simulink model "testTurtleBotModel"  (R2019b)
settings: Solver=FixedStepAuto  StartTime=0.0  StopTime=inf  FixedStep=sampleTime  RelTol=1e-3
PreLoadFcn:
  | linVel = 0;
  | angVel = 0;
  | sampleTime = 0.25;
  | connectToRobot;
InitFcn:
  | close all;
model workspace (MAT data in the model file):
  SL_ROS_VariableLengthArrays_MaxSizes.CommonInfo.ArrayTruncateAction = 'EmitWarning'
  SL_ROS_VariableLengthArrays_MaxSizes.MsgTypeMap = containers.Map
  SL_ROS_VariableLengthArrays_MaxSizes.MsgTypeMap.serialization.keys = {'sensor_msgs/CompressedImage', 'sensor_msgs/Image', 'sensor_msgs/LaserScan', 'sensor_msgs/PointCloud2'}
  SL_ROS_VariableLengthArrays_MaxSizes.MsgTypeMap.serialization.values{1}(1).PropertyName = 'Data'
  SL_ROS_VariableLengthArrays_MaxSizes.MsgTypeMap.serialization.values{1}(1).DataType = 'uint8'
  SL_ROS_VariableLengthArrays_MaxSizes.MsgTypeMap.serialization.values{1}(1).MaxLength = 6220800
  SL_ROS_VariableLengthArrays_MaxSizes.MsgTypeMap.serialization.values{1}(2).PropertyName = 'Format'
  SL_ROS_VariableLengthArrays_MaxSizes.MsgTypeMap.serialization.values{1}(2).DataType = 'uint8'
  SL_ROS_VariableLengthArrays_MaxSizes.MsgTypeMap.serialization.values{1}(2).MaxLength = 128
  SL_ROS_VariableLengthArrays_MaxSizes.MsgTypeMap.serialization.values{2}(1).PropertyName = 'Data'
  SL_ROS_VariableLengthArrays_MaxSizes.MsgTypeMap.serialization.values{2}(1).DataType = 'uint8'
  SL_ROS_VariableLengthArrays_MaxSizes.MsgTypeMap.serialization.values{2}(1).MaxLength = 921600
  SL_ROS_VariableLengthArrays_MaxSizes.MsgTypeMap.serialization.values{2}(2).PropertyName = 'Encoding'
  SL_ROS_VariableLengthArrays_MaxSizes.MsgTypeMap.serialization.values{2}(2).DataType = 'uint8'
  SL_ROS_VariableLengthArrays_MaxSizes.MsgTypeMap.serialization.values{2}(2).MaxLength = 128
  SL_ROS_VariableLengthArrays_MaxSizes.MsgTypeMap.serialization.values{3}(1).PropertyName = 'Intensities'
  SL_ROS_VariableLengthArrays_MaxSizes.MsgTypeMap.serialization.values{3}(1).DataType = 'single'
  SL_ROS_VariableLengthArrays_MaxSizes.MsgTypeMap.serialization.values{3}(1).MaxLength = 640
  SL_ROS_VariableLengthArrays_MaxSizes.MsgTypeMap.serialization.values{3}(2).PropertyName = 'Ranges'
  SL_ROS_VariableLengthArrays_MaxSizes.MsgTypeMap.serialization.values{3}(2).DataType = 'single'
  SL_ROS_VariableLengthArrays_MaxSizes.MsgTypeMap.serialization.values{3}(2).MaxLength = 640
  SL_ROS_VariableLengthArrays_MaxSizes.MsgTypeMap.serialization.values{4}(1).PropertyName = 'Data'
  SL_ROS_VariableLengthArrays_MaxSizes.MsgTypeMap.serialization.values{4}(1).DataType = 'uint8'
  SL_ROS_VariableLengthArrays_MaxSizes.MsgTypeMap.serialization.values{4}(1).MaxLength = 66355200
  SL_ROS_VariableLengthArrays_MaxSizes.MsgTypeMap.serialization.values{4}(2).PropertyName = 'Fields'
  SL_ROS_VariableLengthArrays_MaxSizes.MsgTypeMap.serialization.values{4}(2).DataType = 'sensor_msgs/PointField'
  SL_ROS_VariableLengthArrays_MaxSizes.MsgTypeMap.serialization.values{4}(2).MaxLength = 16
  SL_ROS_VariableLengthArrays_MaxSizes.MsgTypeMap.serialization.uniformity = 0
  SL_ROS_VariableLengthArrays_MaxSizes.MsgTypeMap.serialization.keyType = 'char'
  SL_ROS_VariableLengthArrays_MaxSizes.MsgTypeMap.serialization.valueType = 'any'
undefined symbols (not defined in the file or in its folder): Angular, Linear
libraries: robotlib x8, robotcorelib x1, visionsinks x1
settings Model: EnablePacing=on  Creator=scastro  LastModifiedBy=scastro
settings SolverCC: AutoInsertRateTranBlk=on
settings DataIOCC: ReturnWorkspaceOutputs=off
settings OptimizationCC: EnhancedBackFolding=on  PassReuseOutputArgsAs=Individual arguments  ZeroExternalMemoryAtStartup=off  ZeroInternalMemoryAtStartup=off  MaxStackSize=64  OptimizeBlockOrder=speed  DifferentSizesBufferReuse=on  OptimizationCustomize=off  EfficientTunableParamExpr=on
settings DebuggingCC: ParameterTunabilityLossMsg=error  ArithmeticOperatorsInVariantConditions=warning
settings HardwareCC: ProdBitPerPointer=32  ProdBitPerSizeT=32  ProdBitPerPtrDiffT=32  ProdLargestAtomicFloat=None  ProdIntDivRoundTo=Undefined  ProdEndianess=Unspecified  ProdWordSize=32  ProdHWDeviceType=Generic->Unspecified (assume 32-bit Generic)
settings SFSimCC: SimUseLocalCustomCode=off  MATLABDynamicMemAlloc=off  CustomCodeUndefinedFunction=UseInterfaceOnly
settings RTWCC: SystemTargetFile=ert.tlc  HardwareBoard=Robot Operating System (ROS)  TLCOptions="-aInlineSetEventsForThisBaseRateFcn=TLC_FALSE -aSuppressMultiTaskScheduler=TLC_FALSE  -aRateBasedStepFcn=0"  TemplateMakefile=ert_default_tmf  GenerateReport=on  RTWUseLocalCustomCode=off  Toolchain=Catkin  IncludeHyperlinkInReport=on  LaunchReport=on  TargetLang=C++  GenerateTraceInfo=on  GenerateTraceReport=on  GenerateTraceReportSl=on  GenerateTraceReportSf=on  GenerateTraceReportEml=on
settings CodeAppCC: ForceParamTrailComments=on  IgnoreCustomStorageClasses=off  OperatorAnnotations=on  SimulinkDataObjDesc=on  SFDataObjDesc=on  InsertBlockDesc=on

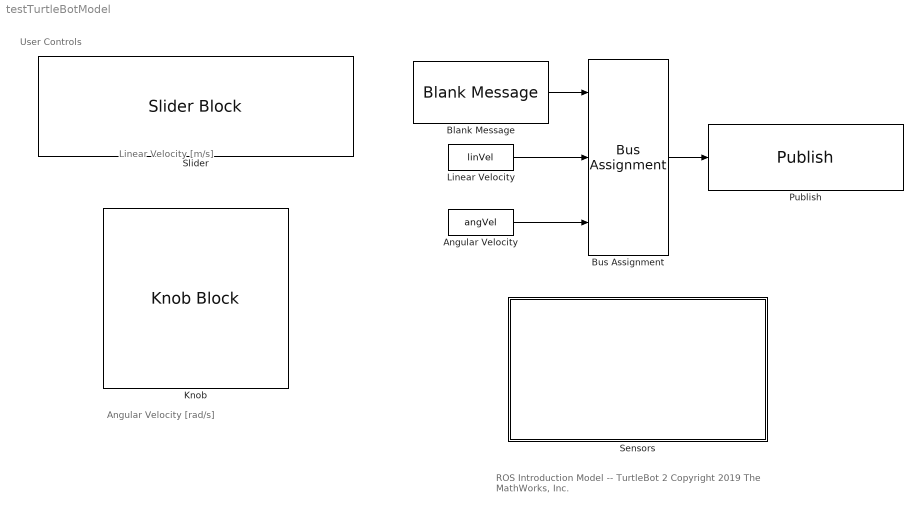
== system testTurtleBotModel ==
  note: User Controls
  note: Linear Velocity [m/s]
  note: Angular Velocity [rad/s]
  note: ROS Introduction Model -- TurtleBot 2
      |
      | Copyright 2019 The MathWorks, Inc.
  Angular Velocity : Constant  Value=angVel
  Blank Message : robotlib/Blank Message  messageClass=Message  entityType=geometry_msgs/Twist  messageType=geometry_msgs/Twist  SampleTime=-1
      settings: SourceProductBaseCode=RO
  Bus Assignment : BusAssignment  AssignedSignals=Linear.X,Angular.Z
  Knob : KnobBlock  ScaleMin=-1  ScaleMax=1  TickInterval=0.25
  Linear Velocity : Constant  Value=linVel
  Publish : robotlib/Publish  topicSource=Select from ROS network  topic=/mobile_base/commands/velocity  messageType=geometry_msgs/Twist  messageQueueLength=1
      settings: SourceProductBaseCode=RO
  Sensors : Subsystem
  Slider : SliderBlock  ScaleMin=-1  ScaleMax=1  TickInterval=0.25
  wires:
  Blank Message/1 -> Bus Assignment/1
  Bus Assignment/1 -> Publish/1
  Linear Velocity/1 -> Bus Assignment/2
  Angular Velocity/1 -> Bus Assignment/3

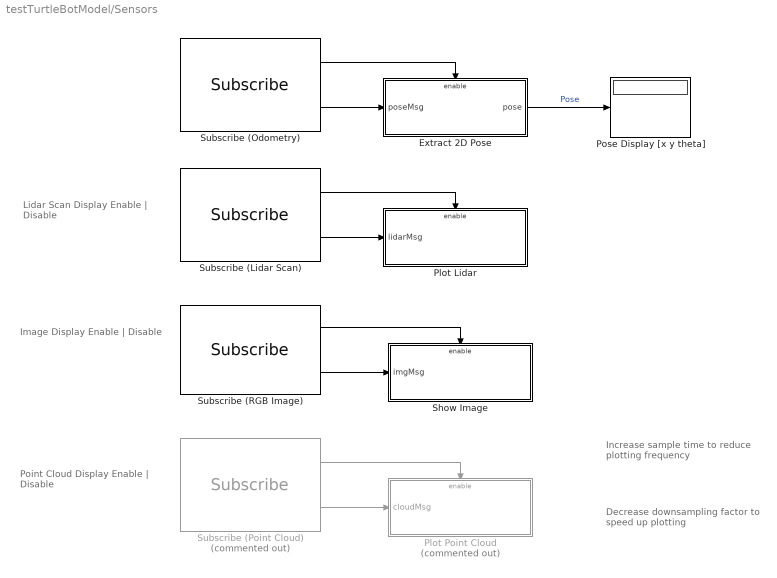
== system testTurtleBotModel/Sensors ==
  note: Increase sample time to reduce plotting frequency
  note: Lidar Scan Display
      | Enable | Disable
  note: Image Display
      | Enable | Disable
  note: Point Cloud Display
      | Enable | Disable
  note: Decrease downsampling factor to speed up plotting
  Extract 2D Pose : Subsystem  TreatAsAtomicUnit=on
  Plot Lidar : Subsystem  TreatAsAtomicUnit=on
  Plot Point Cloud : Subsystem  Commented=on  TreatAsAtomicUnit=on
  Pose Display [x y theta] : Display
  Show Image : Subsystem  TreatAsAtomicUnit=on
  Subscribe (Lidar Scan) : robotlib/Subscribe  topicSource=Select from ROS network  topic=/scan  messageType=sensor_msgs/LaserScan  sampleTime=-1  messageQueueLength=1
      settings: SourceProductBaseCode=RO
  Subscribe (Odometry) : robotlib/Subscribe  topicSource=Select from ROS network  topic=/odom  messageType=nav_msgs/Odometry  sampleTime=-1  messageQueueLength=1
      settings: SourceProductBaseCode=RO
  Subscribe (Point Cloud) : robotlib/Subscribe  Commented=on  topicSource=Select from ROS network  topic=/camera/depth/points  messageType=sensor_msgs/PointCloud2  sampleTime=5  messageQueueLength=1
      settings: SourceProductBaseCode=RO
  Subscribe (RGB Image) : robotlib/Subscribe  topicSource=Select from ROS network  topic=/camera/rgb/image_color  messageType=sensor_msgs/Image  sampleTime=-1  messageQueueLength=1
      settings: SourceProductBaseCode=RO
  wires:
  Extract 2D Pose/1(pose) -> Pose Display [x y theta]/1  "Pose"
  Subscribe (Odometry)/1 -> Extract 2D Pose/Enable
  Subscribe (Odometry)/2 -> Extract 2D Pose/1(poseMsg)
  Subscribe (RGB Image)/2 -> Show Image/1(imgMsg)
  Subscribe (RGB Image)/1 -> Show Image/Enable
  Subscribe (Point Cloud)/2 -> Plot Point Cloud/1(cloudMsg)
  Subscribe (Point Cloud)/1 -> Plot Point Cloud/Enable
  Subscribe (Lidar Scan)/2 -> Plot Lidar/1(lidarMsg)
  Subscribe (Lidar Scan)/1 -> Plot Lidar/Enable

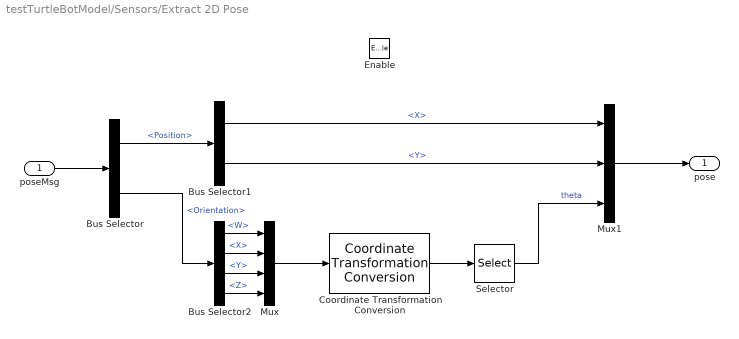
== system testTurtleBotModel/Sensors/Extract 2D Pose ==
  poseMsg : Inport
  Enable : EnablePort
  Bus Selector : BusSelector  OutputSignals=Pose.Pose.Position,Pose.Pose.Orientation
  Bus Selector1 : BusSelector  OutputSignals=X,Y
  Bus Selector2 : BusSelector  OutputSignals=W,X,Y,Z
  Coordinate Transformation Conversion : robotcorelib/Coordinate Transformation Conversion  InputRepresentation=Quaternion  InputEulerSequence=ZYX  ShowTrVecInputPort=on  OutputRepresentation=Euler Angles  OutputEulerSequence=ZYX  ShowTrVecOutputPort=on  SimulateUsing=Interpreted execution
      settings: SourceProductBaseCode=RO
  Mux : Mux
  Mux1 : Mux  Inputs=3
  Selector : Selector  InputPortWidth=3  IndexOptions=Index vector (dialog)  Indices=1  OutputSizes=1
  pose : Outport  VectorParamsAs1DForOutWhenUnconnected=off
  wires:
  poseMsg/1 -> Bus Selector/1
  Bus Selector/1 -> Bus Selector1/1  "<Position>"
  Bus Selector/2 -> Bus Selector2/1  "<Orientation>"
  Bus Selector2/1 -> Mux/1  "<W>"
  Bus Selector2/2 -> Mux/2  "<X>"
  Bus Selector2/3 -> Mux/3  "<Y>"
  Bus Selector2/4 -> Mux/4  "<Z>"
  Coordinate Transformation Conversion/1 -> Selector/1
  Mux/1 -> Coordinate Transformation Conversion/1
  Mux1/1 -> pose/1
  Selector/1 -> Mux1/3  "theta"
  Bus Selector1/2 -> Mux1/2  "<Y>"
  Bus Selector1/1 -> Mux1/1  "<X>"

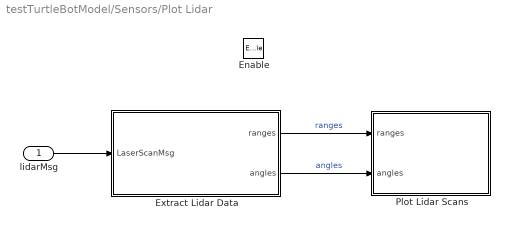
== system testTurtleBotModel/Sensors/Plot Lidar ==
  lidarMsg : Inport
  Enable : EnablePort  PropagateVarSize=During execution
  Extract Lidar Data : MATLAB Function  TreatAsAtomicUnit=on  mask(Extract Range Data){angLimits=[-pi/2 pi/2], rangeLimits=[0 5], numScans=640}
      mask prompts: angLimits "Min and Max Angles [rad]"; rangeLimits "Min and Max Ranges [m]"; numScans "Maximum Number of Scans"
  Plot Lidar Scans : MATLAB Function  InitFcn=clear lidarPlotHelper  TreatAsAtomicUnit=on
  wires:
  lidarMsg/1 -> Extract Lidar Data/1(LaserScanMsg)
  Extract Lidar Data/2(angles) -> Plot Lidar Scans/2(angles)  "angles"
  Extract Lidar Data/1(ranges) -> Plot Lidar Scans/1(ranges)  "ranges"

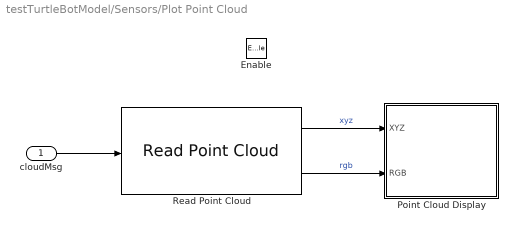
== system testTurtleBotModel/Sensors/Plot Point Cloud ==
  cloudMsg : Inport
  Enable : EnablePort
  Point Cloud Display : MATLAB Function  TreatAsAtomicUnit=on  mask(Point Cloud Display){xLim=[-2 2], yLim=[-0.5 2], zLim=[-0.5 5], sampleFactor=0.02}
      mask prompts: xLim "X Limits [m]"; yLim "Y Limits [m]"; zLim "Z Limits [m]"; sampleFactor "Downsample Factor"
      mask help: Displays a point cloud using the Computer Vision System Toolbox "pcplayer"
  Read Point Cloud : robotlib/Read Point Cloud  MaximumPointCloudSize=[1080, 1920]  PreserveStructure=off  ShowRGBOutput=on  ShowIntensityOutput=off  ShowErrorCodeOutput=off  VariableSizeOutputs=off
      settings: SourceProductName=Robotics System Toolbox  SourceProductBaseCode=RO
  wires:
  cloudMsg/1 -> Read Point Cloud/1
  Read Point Cloud/1 -> Point Cloud Display/1(XYZ)  "xyz"
  Read Point Cloud/2 -> Point Cloud Display/2(RGB)  "rgb"

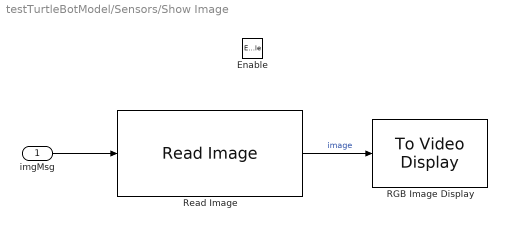
== system testTurtleBotModel/Sensors/Show Image ==
  imgMsg : Inport
  Enable : EnablePort
  RGB Image Display : visionsinks/To Video Display  windowSizeMode=Normal  openAtMdlStart=on  fullScreen=off  videoWindowX=1036  videoWindowY=102  saveWindowSize=off  videoWindowWidth=689  videoWindowHeight=510  inputColorFormat=RGB  inputType=Obsolete  imagePorts=One multidimensional signal  OutputDevice=On-screen video monitor  dataOrg=Column-major  isWindowOpen=off
      settings: SourceProductName=Computer Vision Toolbox
  Read Image : robotlib/Read Image  MaximumImageSize=[480, 640]  ImageEncoding=bgr8  ShowAlphaOutput=off  ShowErrorCodeOutput=off  VariableSizeOutputs=off
      settings: SourceProductName=Robotics System Toolbox  SourceProductBaseCode=RO
  wires:
  imgMsg/1 -> Read Image/1
  Read Image/1 -> RGB Image Display/1  "image"

== matlab function testTurtleBotModel/Sensors/Plot Lidar/Extract Lidar Data ==
  data: LaserScanMsg input; ranges output size=numScans; angles output size=numScans; angLimits parameter; rangeLimits parameter
function [ranges,angles] = ExtractRangeData(LaserScanMsg, angLimits, rangeLimits)
%#codegen

% Extract Range information
rawRanges = double(LaserScanMsg.Ranges);

% Construct Angles vector using AngleMin and AngleIncrement from sensor
% reading.
angMin = double(LaserScanMsg.AngleMin);
angIncrement = double(LaserScanMsg.AngleIncrement);

numReadings = numel(rawRanges);
rawAngles = angMin + (0:numReadings-1)' * angIncrement;

% Wrap the angles to the (-pi,pi] interval.
anglesWrapped = robotics.internal.wrapToPi(double(rawAngles));

% Filter the angles by angle and range limits
indices = (anglesWrapped >= angLimits(1)) & (anglesWrapped <= angLimits(2)) & ...
          (rawRanges >= rangeLimits(1)) & (rawRanges <= rangeLimits(2));
angles = anglesWrapped(indices);
ranges = rawRanges(indices);

== matlab function testTurtleBotModel/Sensors/Plot Point Cloud/Point Cloud Display ==
  data: XYZ input; RGB input; xLim parameter; yLim parameter; zLim parameter; sampleFactor parameter
function plotPtCloud(XYZ, RGB, xLim, yLim, zLim, sampleFactor)
% PLOTPTCLOUD Displays point cloud messages in a pcplayer

coder.extrinsic('pcplayer');
coder.extrinsic('pointCloud');
coder.extrinsic('pcdownsample');
persistent player
if isempty(player)
   player = pcplayer(xLim,yLim,zLim, ...
            'VerticalAxis','Y','VerticalAxisDir','Down');
end

if ~isempty(XYZ)
    ptCloud = pointCloud(XYZ,'Color',RGB);
    ptCloud = pcdownsample(ptCloud,'random',sampleFactor);
    view(player,ptCloud);
end

== matlab function testTurtleBotModel/Sensors/Plot Lidar/Plot Lidar Scans ==
  data: ranges input; angles input
function plotLidar(ranges,angles)

% Call the lidarPlotHelper function as interpreted
coder.extrinsic('lidarPlotHelper');
lidarPlotHelper(ranges,angles);

end
